simulink model "model"  (R2020b)
settings: Solver=FixedStepAuto  StartTime=0.0  StopTime=10.0  FixedStep=0.5  RelTol=1e-3
libraries: SignalEditorBlockLib x1
settings Model: Creator=Arvind Hishikar  LastModifiedBy=Arvind Hishikar

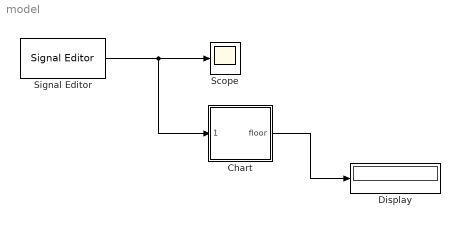
== system model ==
  Chart : Stateflow chart  TreatAsAtomicUnit=on
  Display : Display
  Scope : Scope
  Signal Editor : SignalEditorBlockLib/Signal Editor  FileName=test.mat  ActiveScenario=Scenario  ActiveSignal=lif  IsBus=off  OutputBusObjectStr=Bus: BusObject  SampleTime=0  Interpolate=off  ZeroCross=off  OutputAfterFinalValue=Setting to zero  Unit=inherit  PreserveSignalName=on
  wires:
  Signal Editor/1 -> Scope/1, Chart/1(lif_data)
  Chart/1(floor) -> Display/1

== stateflow chart model/Chart ==
  state disp_floor_number
    state down
    state idle
    state up
      exit:
      floor=floor_count;
    (default) -> idle
    down -> idle : [lif_data==0]
    idle -> up [order 1] : [lif_data==1]{floor_count=floor_count+1}
    idle -> down [order 2] : [lif_data==-1]{floor_count=floor_count-1}
    up -> idle : [lif_data==0]
  (default) -> disp_floor_number
  data: lif_data input; floor output; floor_count local =0
